simulink model "exp2simulink"  (R2017a)
settings: Solver=ode1  StartTime=0.0  StopTime=27  FixedStep=0.01  RelTol=1e-3
values from neighbouring files (symbols this model uses):
  K = KKt/Kt    [exp1analise.m]
  Kp = 1.38    [exp1analise.m]
  Kt = p1(1)    [exp1analise.m]
  T = 0.25    [exp1analise.m]
settings Model: Creator=zolubas  LastModifiedBy=zolubas
settings SolverCC: ZeroCrossControl=EnableAll
settings DataIOCC: SaveFormat=Array  SaveOutput=off  TimeSaveName=tsim

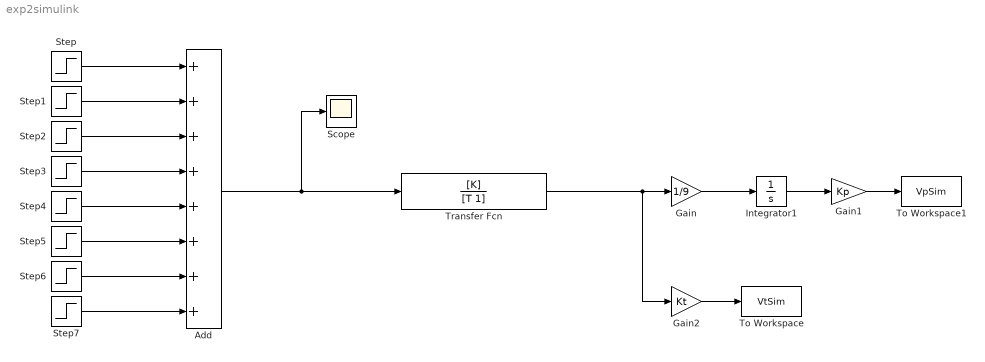
== system exp2simulink ==
  Add : Sum  Inputs=++++++++
  Gain : Gain  Gain=1/9
  Gain1 : Gain  Gain=Kp
  Gain2 : Gain  Gain=Kt
  Integrator1 : Integrator
  Scope : Scope
  Step : Step  SampleTime=0
  Step1 : Step  Time=4  After=-2  SampleTime=0
  Step2 : Step  Time=7  After=3  SampleTime=0
  Step3 : Step  Time=10  After=-4  SampleTime=0
  Step4 : Step  Time=13  After=5  SampleTime=0
  Step5 : Step  Time=16  After=-6  SampleTime=0
  Step6 : Step  Time=19  After=7  SampleTime=0
  Step7 : Step  Time=22  After=-8  SampleTime=0
  To Workspace : ToWorkspace  VariableName=VtSim  SampleTime=-1
  To Workspace1 : ToWorkspace  VariableName=VpSim  SampleTime=-1
  Transfer Fcn : TransferFcn  Numerator=[K]  Denominator=[T 1]
  wires:
  Add/1 -> Scope/1, Transfer Fcn/1
  Transfer Fcn/1 -> Gain2/1, Gain/1
  Gain2/1 -> To Workspace/1
  Step/1 -> Add/1
  Step1/1 -> Add/2
  Step2/1 -> Add/3
  Step3/1 -> Add/4
  Step4/1 -> Add/5
  Step5/1 -> Add/6
  Step6/1 -> Add/7
  Step7/1 -> Add/8
  Gain1/1 -> To Workspace1/1
  Gain/1 -> Integrator1/1
  Integrator1/1 -> Gain1/1
